simulink model "sim_dlqr"  (R2020a)
settings: Solver=VariableStepAuto  StartTime=0.0  StopTime=10.0  RelTol=1e-3
libraries: simulink x1
settings Model: Creator=10853  LastModifiedBy=yztk

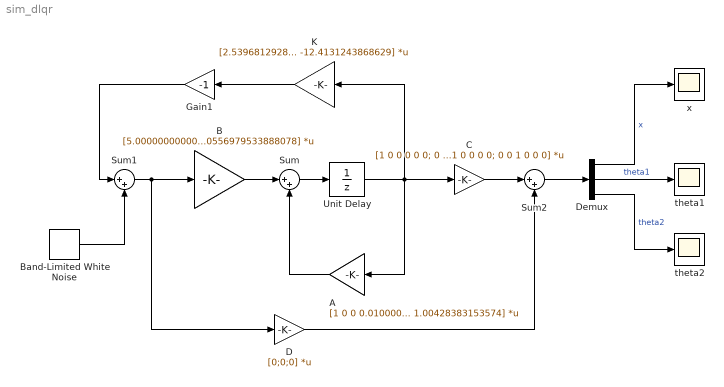
== system sim_dlqr ==
  A : Gain  Gain=|  Multiplication=Matrix(K*u)
      | [1	0	0	0.0100000000000000	0	0
      | 0	1.00948527764292	-0.00586000227576607	0	0.0100315917459796	-1.95154647198305e-05
      | 0	-0.00455406549794487	1.00428383153574	0	-1.51663259457220e-05	0.0100142694595334
      | 0	0	0	1	0	0
      | 0	1.90093431499086	-1.17468318519198	0	1.00948527764292	-0.00586000227576607
      | 0	-0.912897967091567	0.858263852890995	0	-0.00455406549794487	1.00428383153574]
  B : Gain  Gain=|  Multiplication=Matrix(K*u)
      | [5.00000000000000e-05;
      | 0.000369909680682630;
      | -2.75493533285270e-05;
      | 0.0100000000000000;
      | 0.0741039725640779;
      | -0.00556979533888078]
  Band-Limited White Noise : simulink/Sources/Band-Limited White Noise  Cov=0  Ts=0.01  seed=[23341]
  C : Gain  Gain=|  Multiplication=Matrix(K*u)
      | [1 0 0 0 0 0;
      | 0 1 0 0 0 0;
      | 0 0 1 0 0 0]
  D : Gain  Gain=[0;0;0]  Multiplication=Matrix(K*u)
  Demux : Demux  Outputs=3
  Gain1 : Gain  Gain=-1
  K : Gain  Gain="[2.53968129287746\t105.510812672320\t-119.103945413954\t3.48266173346965\t3.96030597261041\t-12.4131243868629]"  Multiplication=Matrix(K*u)
  Sum : Sum  Inputs=|++
  Sum1 : Sum  Inputs=|++
  Sum2 : Sum  Inputs=|++
  Unit Delay : UnitDelay  InitialCondition=[0 5*pi/180 5*pi/180 0 0 0]  SampleTime=0.01  HasFrameUpgradeWarning=on
  theta1 : Scope
  theta2 : Scope
  x : Scope
  wires:
  B/1 -> Sum/1
  Sum/1 -> Unit Delay/1
  A/1 -> Sum/2
  Unit Delay/1 -> K/1, A/1, C/1
  Demux/1 -> x/1  "x"
  Demux/2 -> theta1/1  "theta1"
  Demux/3 -> theta2/1  "theta2"
  K/1 -> Gain1/1
  Gain1/1 -> Sum1/1
  Band-Limited White Noise/1 -> Sum1/2
  D/1 -> Sum2/2
  Sum1/1 -> D/1, B/1
  Sum2/1 -> Demux/1
  C/1 -> Sum2/1
